simulink model "PID_IDEAL_Kp_Ki_Kd_r2009a"  (Simulink 7.6)
settings: Solver=ode3  StartTime=0.0  StopTime=Tmax  FixedStep=0.001  RelTol=1e-3
values from neighbouring files (symbols this model uses):
  A = 1    [script_exemplo_simulink.m]
  K = 2    [script_exemplo_simulink.m]
  Kd = 0    [script_exemplo_simulink.m]
  Ki = 0    [script_exemplo_simulink.m]
  Kp = 1    [script_exemplo_simulink.m]
  Tau = 4    [script_exemplo_simulink.m]
  teta = 1    [script_exemplo_simulink.m]
settings Model: Creator=Marcos  LastModifiedBy=Administrador
settings DataIOCC: LimitDataPoints=off
settings DebuggingCC: StrictBusMsg=Warning

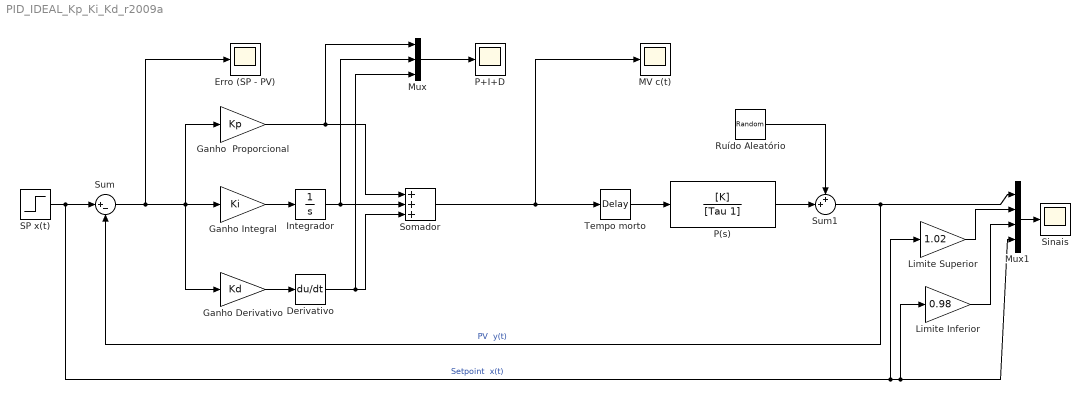
== system PID_IDEAL_Kp_Ki_Kd_r2009a ==
  Derivativo : Derivative
  Erro (SP - PV) : Scope
      settings: TimeRange=10  YMin=0.2  YMax=1  SaveName=Erro  DataFormat=Array
  Ganho Derivativo : Gain  Gain=Kd
  Ganho Integral : Gain  Gain=Ki
  Ganho  Proporcional : Gain  Gain=Kp
  Integrador : Integrator
  Limite Inferior : Gain  Gain=0.98
  Limite Superior : Gain  Gain=1.02
  MV c(t) : Scope
      settings: TimeRange=10  YMin=0.2  YMax=1  SaveName=MV  DataFormat=Array
  Mux : Mux  Inputs=3
  Mux1 : Mux
  P(s) : TransferFcn  Numerator=[K]  Denominator=[Tau 1]
  P+I+D : Scope
      settings: TimeRange=10  YMin=0  YMax=1  SaveName=SINAIS_PID  DataFormat=Array
  Ruído Aleatório : RandomNumber  Variance=0  SampleTime=0
  SP x(t) : Step  Time=0  After=A  SampleTime=0
  Sinais : Scope
      settings: TimeRange=15  YMin=0  YMax=1.4  SaveName=Sinais  DataFormat=Array
  Somador : Sum  Inputs=+++
  Sum : Sum  Inputs=|+-
  Sum1 : Sum  Inputs=++|
  Tempo morto : TransportDelay  DelayTime=teta
  wires:
  SP x(t)/1 -> Sum/1, Mux1/4, Limite Inferior/1, Limite Superior/1  "Setpoint  x(t)"
  Sum/1 -> Erro (SP - PV)/1, Ganho Derivativo/1, Ganho  Proporcional/1, Ganho Integral/1
  P(s)/1 -> Sum1/2
  Sum1/1 -> Sum/2, Mux1/1  "PV  y(t)"
  Ruído Aleatório/1 -> Sum1/1
  Mux1/1 -> Sinais/1
  Ganho  Proporcional/1 -> Mux/1, Somador/1
  Mux/1 -> P+I+D/1
  Ganho Integral/1 -> Integrador/1
  Ganho Derivativo/1 -> Derivativo/1
  Integrador/1 -> Somador/2, Mux/2
  Derivativo/1 -> Mux/3, Somador/3
  Tempo morto/1 -> P(s)/1
  Somador/1 -> Tempo morto/1, MV c(t)/1
  Limite Inferior/1 -> Mux1/3
  Limite Superior/1 -> Mux1/2
